simulink model "kalmanext"  (R2015b)
settings: Solver=FixedStepDiscrete  StartTime=0.0  StopTime=10  FixedStep=T  RelTol=1e-3
InitFcn:
  | param
values from neighbouring files (symbols this model uses):
  T = 0.1    [param.m]
undefined symbols (not defined in the file or in its folder): DiscIntNeverNeededParam
libraries: commchan3 x2, simulink x1
settings Model: Creator=mishuk  LastModifiedBy=mishuk
settings DataIOCC: SaveFormat=Array
settings OptimizationCC: ExpressionDepthLimit=2147483647
settings DebuggingCC: UnderspecifiedInitializationDetection=Classic  MergeDetectMultiDrivingBlocksExec=none  SolverPrmCheckMsg=warning  StateNameClashWarn=warning
settings HardwareCC: ProdBitPerPointer=32  ProdLargestAtomicFloat=None  ProdIntDivRoundTo=Undefined  ProdEndianess=Unspecified  ProdWordSize=32  ProdHWDeviceType=32-bit Generic
settings RTWCC: GenCodeOnly=on
settings GRTTargetCC: GeneratePreprocessorConditionals=Disable all
settings ConfigComp: CovModelRefEnable=Off

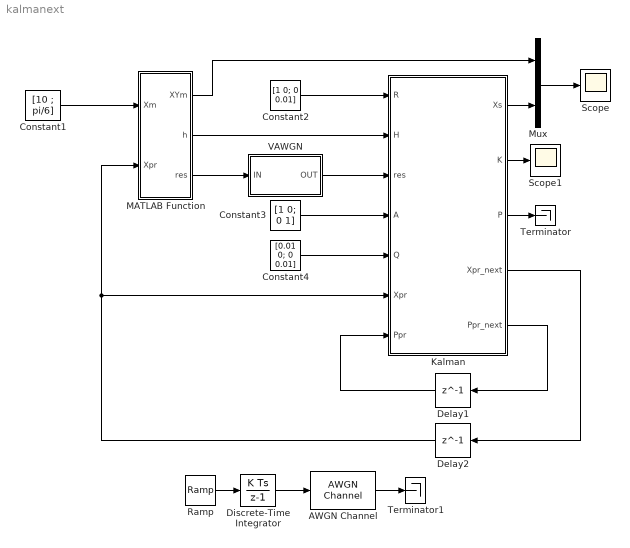
== system kalmanext ==
  AWGN Channel : commchan3/AWGN Channel  InputProcessing=Columns as channels (frame based)  seed=67  noiseMode=Variance from mask  EbNodB=10  EsNodB=10  SNRdB=10  bitsPerSym=1  Ps=1  Tsym=1  variance=noiseVariance
  Constant1 : Constant  Value=[10 ; pi/6]  VectorParams1D=off  SampleTime=-1
  Constant2 : Constant  Value=[1 0; 0 0.01]  SampleTime=-1
  Constant3 : Constant  Value=[1 0; 0 1]  SampleTime=-1
  Constant4 : Constant  Value=[0.01 0; 0 0.01]  SampleTime=-1
  Delay1 : Delay  DelayLength=1  InitialCondition=eye(2)
  Delay2 : Delay  DelayLength=1  InitialCondition=[1; 1]
  Discrete-Time Integrator : DiscreteIntegrator  gainval=1  InitialConditionSetting=State (most efficient)  SampleTime=T  ICPrevOutput=DiscIntNeverNeededParam  ICPrevScaledInput=DiscIntNeverNeededParam
  Kalman : MATLAB Function  TreatAsAtomicUnit=on
  MATLAB Function : MATLAB Function  TreatAsAtomicUnit=on
  Mux : Mux  Inputs=2
  Ramp : simulink/Sources/Ramp  slope=1  start=0  X0=0
  Scope : Scope
  Scope1 : Scope
  Terminator : Terminator
  Terminator1 : Terminator
  VAWGN : Subsystem
  wires:
  Kalman/5(Ppr_next) -> Delay1/1
  Delay1/1 -> Kalman/7(Ppr)
  Kalman/4(Xpr_next) -> Delay2/1
  Delay2/1 -> Kalman/6(Xpr), MATLAB Function/2(Xpr)
  Kalman/3(P) -> Terminator/1
  MATLAB Function/2(h) -> Kalman/2(H)
  Constant2/1 -> Kalman/1(R)
  Constant3/1 -> Kalman/4(A)
  Mux/1 -> Scope/1
  Constant4/1 -> Kalman/5(Q)
  Ramp/1 -> Discrete-Time Integrator/1
  MATLAB Function/1(XYm) -> Mux/1
  AWGN Channel/1 -> Terminator1/1
  Discrete-Time Integrator/1 -> AWGN Channel/1
  Kalman/2(K) -> Scope1/1
  Kalman/1(Xs) -> Mux/2
  Constant1/1 -> MATLAB Function/1(Xm)
  MATLAB Function/3(res) -> VAWGN/1(IN)
  VAWGN/1(OUT) -> Kalman/3(res)

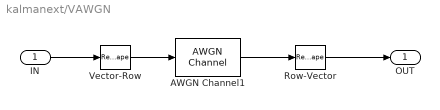
== system kalmanext/VAWGN ==
  IN : Inport
  AWGN Channel1 : commchan3/AWGN Channel  InputProcessing=Columns as channels (frame based)  seed=67  noiseMode=Variance from mask  EbNodB=10  EsNodB=10  SNRdB=10  bitsPerSym=1  Ps=1  Tsym=1  variance=[1; 0.01]
  Row-Vector : Reshape  OutputDimensionality=Customize  OutputDimensions=[2,1]
  Vector-Row : Reshape  OutputDimensionality=Customize  OutputDimensions=[1,2]
  OUT : Outport
  wires:
  IN/1 -> Vector-Row/1
  Vector-Row/1 -> AWGN Channel1/1
  AWGN Channel1/1 -> Row-Vector/1
  Row-Vector/1 -> OUT/1

== matlab function kalmanext/MATLAB Function ==
  data: XYm output; Xm input; Xpr input; h output; res output
function [XYm, h, res] = H(Xm, Xpr)
%#codegen

[Bpr, Rpr] = cart2pol(Xpr(1), Xpr(2));
[xm, ym] = pol2cart(Xm(2), Xm(1));
h = [Xpr(1) Xpr(2) ; -Xpr(2)/Rpr Xpr(1)/Rpr] / Rpr;
res = Xm - [Rpr; Bpr];
XYm = [xm; ym];

== matlab function kalmanext/Kalman ==
  data: Xs output; R input; H input; res input; A input; Q input; Xpr input; K output; Ppr input; P output; Xpr_next output; Ppr_next output
function [Xs, K, P, Xpr_next, Ppr_next] = kalmanext(R, H, res, A, Q, Xpr, Ppr)

%% estimation
K = Ppr*H'*(R+H*Ppr*H')^(-1);
Xs = Xpr + K*res;
I = eye(length(Xpr));
P = (I - K*H)*Ppr*(I-K*H)' + K*R*(K');

%% prediction
Xpr_next = A*Xs;
Ppr_next = A*P*A' + Q;
